simulink subsystem "thermal_basic_peripherals"  (R2023a)
settings: Solver=VariableStepAuto  StartTime=0.0  StopTime=10.0  RelTol=1e-3
values from neighbouring files (symbols this model uses):
  coolant_initial_pressure = 0.111325    [thermal_plant_h2f175_parameters.m]
  coolant_initial_temperature = 293.15    [thermal_plant_h2f175_parameters.m]
  coolant_tube_D = 0.05    [thermal_plant_h2f175_parameters.m]
  tcp_time_constant = 2    [thermal_plant_h2f175_parameters.m]
undefined symbols (not defined in the file or in its folder): air_cp, air_HC_min, air_HC_nom, air_rho, air_vel_nom, radiator_area_air, radiator_area_fins, radiator_area_primary, radiator_n_tubes, radiator_tube_height, radiator_tube_length, radiator_width
libraries: fl_lib x30, nesl_utility x20, SimscapeFluids_lib x5
settings Model: Creator=stefan.notter  LastModifiedBy=stefan.notter

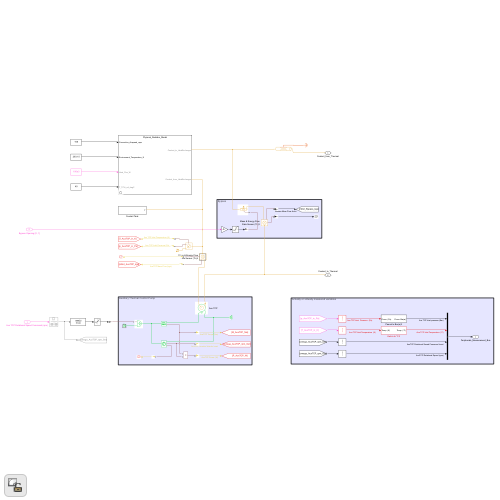
[thumbnail: Simulink's stored preview of the top-level diagram]
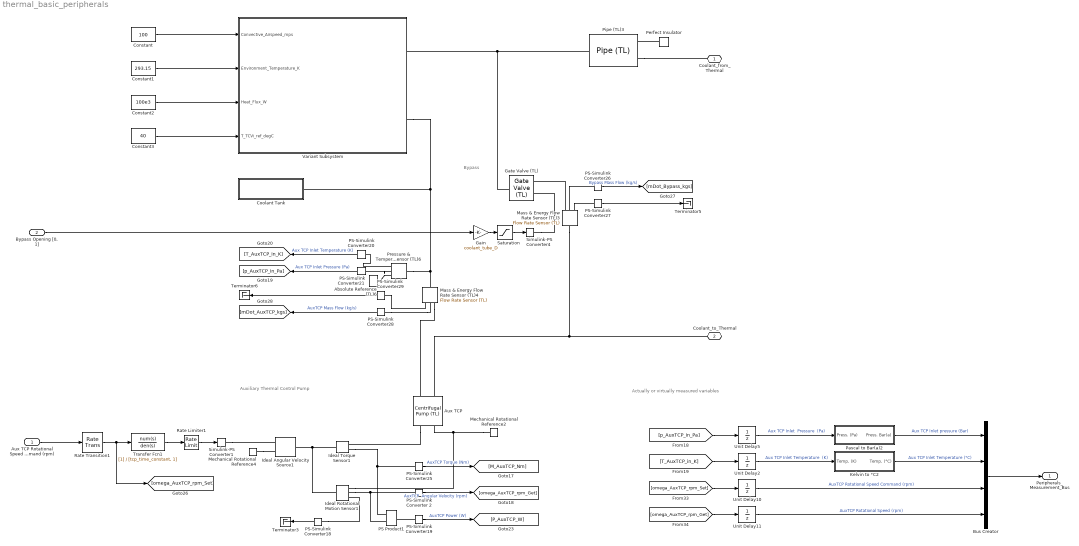
== system thermal_basic_peripherals ==
  note: Auxiliary Thermal Control Pump
  note: Actually or virtually measured variables
  note: Bypass
  Aux TCP Rotational Speed Command (rpm) : Inport
  "Bypass Opening [0, 1]" : Inport  Port=2
  Absolute Reference (TL)6 : fl_lib/Thermal Liquid/Elements/Absolute Reference (TL)
  Aux TCP : SimscapeFluids_lib/Thermal Liquid/Pumps & Motors/Centrifugal Pump (TL)  pump_parameterization=fluids.thermal_liquid.pumps_motors.enum.CentrifugalPumpParameterization.Nominal  capacity_ref_nominal=6000/60 lpm  head_ref_nominal=|  power_ref_nominal=0.3 kW  head_ref_max=|  capacity_ref_max=12000/60 lpm  omega_ref_analytic=3500 rpm  flow_rate_1D_TLU=[1000, 2000, 3000, 4000, 5000, 6000, 7000, 8000, 9000, 1000] lpm  head_1D_TLU=[50, 47.5, 45, 40, 35, 25] m  power_1D_TLU=[.6, .75, .85, .93, .98, .99] kW  omega_ref_1D=3500 rpm  rho_ref_1D=998.21 kg/m^3  omega_threshold_factor=1e-2  flow_rate_2D_TLU=[16.67, 23.33, 30, 40, 53.33, 60] lpm  omega_2D_TLU=[2450, 2800, 3150, 3500] rpm  head_2D_TLU=[25, 32.7, 42.5, 50; 24, 31.7, 41, 49; 22.7, 30.5, 39, 47.5; 20, 28, 36, 45; 15.7, 24, 32, 40; 12.5, 21, 29.5, 37.5] m  power_2D_TLU=[.28, .38, .5, .6; .31, .41, .55, .68; .33, .44, .6, .75; .36, .48, .65, .83; .38, .53, .72, .93; .39, .55, .75, .97] kW  rho_ref_2D=998.21 kg/m^3  diameter_ratio=1  mech_orientation=fluids.thermal_liquid.pumps_motors.enum.CentrifugalPumpMechOrientation.Positive  area=9.6211275016187417927918453612935e-4 m^2
      head_ref_nominal=|
      | 1.2*10^5/(1000*9.81)
      |  m
      head_ref_max=|
      | 1.55*10^5/(1000*9.81)
      |  m
      settings: InternalSimscapePortConfiguration="{\"Bottom\":[],\"Left\":[{\"id\":\"A\",\"label\":\"A\",\"type\":\"foundation.thermal_liquid.thermal_liquid\"},{\"id\":\"B\",\"label\":\"B\",\"type\":\"foundation.thermal_liquid.thermal_liquid\"}],\"Right\":[{\"id\":\"R\",\"label\":\"R\",\"type\":\"foundation.mechanical.rotational.rotational\"},{\"id\":\"C\",\"label\":\"C\",\"type\":\"foundation.mechanical.rotational.rotational\"}],\"Top\":[]}"
  Bus Creator : BusCreator  Inputs=4
  Constant : Constant  Value=100
  Constant1 : Constant  Value=293.15
  Constant2 : Constant  Value=100e3
  Constant3 : Constant  Value=40
  Coolant Tank : Subsystem  Tag=PublishSubsystem  mask(Coolant Tank){A=1, x_init=0.08}
      mask prompts: A "Tank area (m^2)"; x_init "Initial coolant level (m)"
      mask help: This subsystem models an expansion tank for the coolant system.
  Gain : Gain  Gain=coolant_tube_D
  Gate Valve (TL) : SimscapeFluids_lib/Thermal Liquid/Valves & Orifices/Flow Control Valves/Gate Valve (TL)  diam_orifice=coolant_tube_D*0.9 m  S_min=0 m  area_leak=1e-12 m^2  smoothing_factor=0.01  area=pi*coolant_tube_D^2/4 m^2  Cd=0.7  Re_c=12
      settings: InternalSimscapePortConfiguration="{\"Bottom\":[],\"Left\":[{\"id\":\"A\",\"label\":\"A\",\"type\":\"foundation.thermal_liquid.thermal_liquid\"},{\"id\":\"S\",\"label\":\"S\",\"type\":\"input\"}],\"Right\":[{\"id\":\"B\",\"label\":\"B\",\"type\":\"foundation.thermal_liquid.thermal_liquid\"}],\"Top\":[]}"
  Ideal Angular Velocity Source1 : fl_lib/Mechanical/Mechanical Sources/Ideal Angular Velocity Source
  Ideal Rotational Motion Sensor1 : fl_lib/Mechanical/Mechanical Sensors/Ideal Rotational Motion Sensor  reference=foundation.enum.MeasurementReference.difference  acceleration_port=false  velocity_port=true  position_port=true  wrap_angle=false  offset=0 rad
  Ideal Torque Sensor1 : fl_lib/Mechanical/Mechanical Sensors/Ideal Torque Sensor
  Kelvin to °C2 : Subsystem
  Mass & Energy Flow Rate Sensor (TL)3 : fl_lib/Thermal Liquid/Sensors/Flow Rate Sensor (TL)  mass_flow_measure=true  volumetric_flow_measure=false  energy_flow_measure=true
      settings: InternalSimscapePortConfiguration="{\"Bottom\":[{\"id\":\"PHI\",\"label\":\"φ\",\"type\":\"output\"}],\"Left\":[{\"id\":\"A\",\"label\":\"A\",\"type\":\"foundation.thermal_liquid.thermal_liquid\"}],\"Right\":[{\"id\":\"B\",\"label\":\"B\",\"type\":\"foundation.thermal_liquid.thermal_liquid\"},{\"id\":\"M\",\"label\":\"M\",\"type\":\"output\"}],\"Top\":[]}"
  Mass & Energy Flow Rate Sensor (TL)4 : fl_lib/Thermal Liquid/Sensors/Flow Rate Sensor (TL)  mass_flow_measure=true  volumetric_flow_measure=false  energy_flow_measure=true
      settings: InternalSimscapePortConfiguration="{\"Bottom\":[{\"id\":\"PHI\",\"label\":\"φ\",\"type\":\"output\"}],\"Left\":[{\"id\":\"A\",\"label\":\"A\",\"type\":\"foundation.thermal_liquid.thermal_liquid\"}],\"Right\":[{\"id\":\"B\",\"label\":\"B\",\"type\":\"foundation.thermal_liquid.thermal_liquid\"},{\"id\":\"M\",\"label\":\"M\",\"type\":\"output\"}],\"Top\":[]}"
  Mechanical Rotational Reference2 : fl_lib/Mechanical/Rotational Elements/Mechanical Rotational Reference
  Mechanical Rotational Reference4 : fl_lib/Mechanical/Rotational Elements/Mechanical Rotational Reference
  PS Product1 : fl_lib/Physical Signals/Functions/PS Product
  PS-Simulink Converter 2 : nesl_utility/PS-Simulink Converter  PhysicalDomain=network_engine_domain  SubClassName=ps_output  LeftPortType=input  RightPortType=output  PseudoPeriodic=off  Frequencies=[]  VectorFormat=1-D array  Unit=rpm  AffineConversion=off
  PS-Simulink Converter{18,20..21,26..29} (7 alike) : nesl_utility/PS-Simulink Converter  PhysicalDomain=network_engine_domain  SubClassName=ps_output  LeftPortType=input  RightPortType=output  PseudoPeriodic=off  Frequencies=[]  VectorFormat=inherit  Unit=inherit  AffineConversion=off
  PS-Simulink Converter19 : nesl_utility/PS-Simulink Converter  PhysicalDomain=network_engine_domain  SubClassName=ps_output  LeftPortType=input  RightPortType=output  PseudoPeriodic=off  Frequencies=[]  VectorFormat=inherit  Unit=W  AffineConversion=off
  PS-Simulink Converter25 : nesl_utility/PS-Simulink Converter  PhysicalDomain=network_engine_domain  SubClassName=ps_output  LeftPortType=input  RightPortType=output  PseudoPeriodic=off  Frequencies=[]  VectorFormat=inherit  Unit=N*m  AffineConversion=off
  Pascal to Bar(a)2 : Subsystem
  Perfect Insulator : fl_lib/Thermal/Thermal Elements/Perfect Insulator  T_specify=off  T_priority=None  T=293.15 K  T_nominal_specify=off  T_nominal_unit=K  T_nominal_value=1
  Pipe (TL)3 : fl_lib/Thermal Liquid/Elements/Pipe (TL)  length=1 m  area=pi*coolant_tube_D^2/4 m^2  Dh=pi*coolant_tube_D*0.9 m  length_add=1 m  roughness=15e-6 m  Re_lam=2000  Re_tur=4000  shape_factor=64  Nu_lam=3.66  dynamic_compressibility=simscape.enum.onoff.on  inertia=simscape.enum.onoff.off  p0=coolant_initial_pressure MPa  T0=coolant_initial_temperature K  mdot0=0 kg/s
  Pressure & Temperature Sensor (TL)6 : fl_lib/Thermal Liquid/Sensors/Pressure & Temperature Sensor (TL)  reference=foundation.enum.MeasurementReference.difference  pressure=true  pressure_spec=foundation.enum.PressureMeasementSpec.Absolute  temperature=true
      settings: InternalSimscapePortConfiguration="{\"Bottom\":[{\"id\":\"T\",\"label\":\"T\",\"type\":\"output\"}],\"Left\":[{\"id\":\"A\",\"label\":\"A\",\"type\":\"foundation.thermal_liquid.thermal_liquid\"}],\"Right\":[{\"id\":\"B\",\"label\":\"B\",\"type\":\"foundation.thermal_liquid.thermal_liquid\"},{\"id\":\"P\",\"label\":\"P\",\"type\":\"output\"}],\"Top\":[]}"
  Rate Limiter1 : RateLimiter  RisingSlewLimit=1000  FallingSlewLimit=-1000  SampleTimeMode=inherited
  Rate Transition1 : RateTransition
  Saturation : Saturate  UpperLimit=coolant_tube_D  LowerLimit=0
  Simulink-PS Converter1 : nesl_utility/Simulink-PS Converter  PhysicalDomain=network_engine_domain  SubClassName=ps_input  LeftPortType=input  RightPortType=output  PseudoPeriodic=off  Frequencies=[]  NoiseDistribution=none  NoiseParameters=[]  Unit=rpm  AffineConversion=off  FilteringAndDerivatives=provide  SimscapeFilterOrder=1  InputFilterTimeConstant=0.001  UdotUserProvided=0
  Simulink-PS Converter4 : nesl_utility/Simulink-PS Converter  PhysicalDomain=network_engine_domain  SubClassName=ps_input  LeftPortType=input  RightPortType=output  PseudoPeriodic=off  Frequencies=[]  NoiseDistribution=none  NoiseParameters=[]  Unit=1  AffineConversion=off  FilteringAndDerivatives=provide  SimscapeFilterOrder=1  InputFilterTimeConstant=0.001  UdotUserProvided=0
  Terminator3 : Terminator
  Terminator5 : Terminator
  Terminator6 : Terminator
  Transfer Fcn1 : TransferFcn  Denominator=[tcp_time_constant, 1]  ContinuousStateAttributes='tcv_opening'
  Unit Delay10 : UnitDelay  SampleTime=-1  HasFrameUpgradeWarning=on
  Unit Delay11 : UnitDelay  SampleTime=-1  HasFrameUpgradeWarning=on
  Unit Delay2 : UnitDelay  InitialCondition=coolant_initial_temperature  SampleTime=-1  HasFrameUpgradeWarning=on
  Unit Delay5 : UnitDelay  InitialCondition=coolant_initial_pressure  SampleTime=-1  HasFrameUpgradeWarning=on
  Variant Subsystem : Subsystem  Variant=on
  Coolant_from_Thermal : PMIOPort  Side=Left
  Coolant_to_Thermal : PMIOPort  Port=2  Side=Left
  Peripherals_Measurement_Bus : Outport
  wires:
  Aux TCP Rotational Speed Command (rpm)/1 -> Rate Transition1/1
  PS-Simulink Converter29/1 -> Terminator6/1
  PS-Simulink Converter20/1 -> [T_AuxTCP_in_K]  "Aux TCP Inlet Temperature (K)"
  PS-Simulink Converter21/1 -> [p_AuxTCP_in_Pa]  "Aux TCP Inlet Pressure (Pa)"
  PS-Simulink Converter19/1 -> [P_AuxTCP_W]  "AuxTCP Power (W)"
  Rate Transition1/1 -> Transfer Fcn1/1, [omega_AuxTCP_rpm_Set]
  PS-Simulink Converter 2/1 -> [omega_AuxTCP_rpm_Get]  "AuxTCP  Angular Velocity (rpm)"
  PS-Simulink Converter25/1 -> [M_AuxTCP_Nm]  "AuxTCP Torque (Nm)"
  PS-Simulink Converter18/1 -> Terminator3/1
  Rate Limiter1/1 -> Simulink-PS Converter1/1
  Transfer Fcn1/1 -> Rate Limiter1/1
  PS-Simulink Converter28/1 -> [mDot_AuxTCP_kgs]  "AuxTCP Mass Flow (kg/s)"
  Pascal to Bar(a)2/1(Press. Bar(a)) -> Bus Creator/1  "Aux TCP Inlet pressure (Bar)"
  Unit Delay10/1 -> Bus Creator/3  "AuxTCP Rotational Speed Command (rpm)"
  Kelvin to °C2/1(Temp. (°C)) -> Bus Creator/2  "Aux TCP Inlet Temperature (°C)"
  [omega_AuxTCP_rpm_Get] -> Unit Delay11/1
  Unit Delay2/1 -> Kelvin to °C2/1(Temp. (K))  "Aux TCP Inlet Temperature  (K)"
  Unit Delay5/1 -> Pascal to Bar(a)2/1(Press. (Pa))  "Aux TCP Inlet  Pressure  (Pa)"
  Unit Delay11/1 -> Bus Creator/4  "AuxTCP Rotational Speed (rpm)"
  [p_AuxTCP_in_Pa] -> Unit Delay5/1
  [T_AuxTCP_in_K] -> Unit Delay2/1
  [omega_AuxTCP_rpm_Set] -> Unit Delay10/1
  Bus Creator/1 -> Peripherals_Measurement_Bus/1
  Constant/1 -> Variant Subsystem/1(Convective_Airspeed_mps)
  Constant1/1 -> Variant Subsystem/2(Environment_Temperature_K)
  Constant2/1 -> Variant Subsystem/3(Heat_Flux_W)
  Constant3/1 -> Variant Subsystem/4(T_TCVi_ref_degC)
  PS-Simulink Converter26/1 -> [mDot_Bypass_kgs]  "Bypass Mass Flow (kg/s)"
  PS-Simulink Converter27/1 -> Terminator5/1
  Gain/1 -> Saturation/1
  "Bypass Opening [0, 1]"/1 -> Gain/1
  Saturation/1 -> Simulink-PS Converter4/1
  connections:
  Mechanical Rotational Reference2/LConn1 -- Aux TCP/RConn2 -- Ideal Rotational Motion Sensor1/RConn1
  Variant Subsystem/RConn2 -- Coolant Tank/RConn1 -- Mass & Energy Flow Rate Sensor (TL)4/LConn1 -- Pressure & Temperature Sensor (TL)6/LConn1
  Ideal Angular Velocity Source1/LConn1 -- Ideal Rotational Motion Sensor1/LConn1 -- Ideal Torque Sensor1/LConn1
  Ideal Rotational Motion Sensor1/RConn2 -- PS Product1/LConn2 -- PS-Simulink Converter 2/LConn1
  Ideal Torque Sensor1/RConn2 -- PS-Simulink Converter25/LConn1 -- PS Product1/LConn1
  Aux TCP/LConn2 -- Coolant_to_Thermal/RConn1 -- Mass & Energy Flow Rate Sensor (TL)3/LConn1
  Gate Valve (TL)/RConn1 -- Variant Subsystem/RConn1 -- Pipe (TL)3/RConn1
  Simulink-PS Converter1/RConn1 -- Ideal Angular Velocity Source1/RConn1
  PS-Simulink Converter28/LConn1 -- Mass & Energy Flow Rate Sensor (TL)4/RConn2
  Pressure & Temperature Sensor (TL)6/RConn1 -- Absolute Reference (TL)6/LConn1
  Pressure & Temperature Sensor (TL)6/RConn2 -- PS-Simulink Converter21/LConn1
  Aux TCP/RConn1 -- Ideal Torque Sensor1/RConn1
  Mechanical Rotational Reference4/LConn1 -- Ideal Angular Velocity Source1/RConn2
  PS-Simulink Converter18/LConn1 -- Ideal Rotational Motion Sensor1/RConn3
  PS-Simulink Converter19/LConn1 -- PS Product1/RConn1
  Mass & Energy Flow Rate Sensor (TL)4/RConn1 -- Aux TCP/LConn1
  Pressure & Temperature Sensor (TL)6/RConn3 -- PS-Simulink Converter20/LConn1
  PS-Simulink Converter29/LConn1 -- Mass & Energy Flow Rate Sensor (TL)4/RConn3
  Mass & Energy Flow Rate Sensor (TL)3/RConn1 -- Gate Valve (TL)/LConn1
  PS-Simulink Converter26/LConn1 -- Mass & Energy Flow Rate Sensor (TL)3/RConn2
  Simulink-PS Converter4/RConn1 -- Gate Valve (TL)/LConn2
  PS-Simulink Converter27/LConn1 -- Mass & Energy Flow Rate Sensor (TL)3/RConn3
  Pipe (TL)3/LConn1 -- Coolant_from_Thermal/RConn1
  Perfect Insulator/LConn1 -- Pipe (TL)3/LConn2

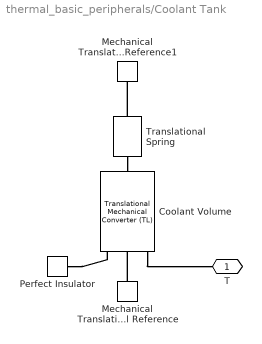
== system thermal_basic_peripherals/Coolant Tank ==
  Coolant Volume : fl_lib/Thermal Liquid/Elements/Translational Mechanical Converter (TL)  mech_orientation=foundation.enum.MechOrientationTranslational.Positive  displacement_spec=foundation.enum.DisplacementSpec.Calculate  x0=x_init m  interface_area=A m^2  dead_volume=A * 0.001 m^3  environment_spec=foundation.enum.pressure_spec.specified  environment_pressure=coolant_initial_pressure MPa  dynamic_compressibility=simscape.enum.onoff.off  p0=env_p MPa  T0=coolant_initial_temperature K
      settings: InternalSimscapePortConfiguration="{\"Bottom\":[],\"Left\":[{\"id\":\"A\",\"label\":\"A\",\"type\":\"foundation.thermal_liquid.thermal_liquid\"},{\"id\":\"C\",\"label\":\"C\",\"type\":\"foundation.mechanical.translational.translational\"},{\"id\":\"H\",\"label\":\"H\",\"type\":\"foundation.thermal.thermal\"}],\"Right\":[{\"id\":\"R\",\"label\":\"R\",\"type\":\"foundation.mechanical.translational.translational\"}],\"Top\":[]}"
  Mechanical Translational Reference : fl_lib/Mechanical/Translational Elements/Mechanical Translational Reference
  Mechanical Translational Reference1 : fl_lib/Mechanical/Translational Elements/Mechanical Translational Reference
  Perfect Insulator : fl_lib/Thermal/Thermal Elements/Perfect Insulator  T_specify=off  T_priority=None  T=0 K  T_nominal_specify=off  T_nominal_unit=K  T_nominal_value=1
  Translational Spring : fl_lib/Mechanical/Translational Elements/Translational Spring  spr_rate=1e6 N/m  v_specify=off  v_priority=None  v=0 m/s  v_nominal_specify=off  v_nominal_unit=m/s  v_nominal_value=1  f_specify=off  f_priority=None  f=0 N  f_nominal_specify=off  f_nominal_unit=N  f_nominal_value=1  x_specify=off  x_priority=High  x=x_init m  x_nominal_specify=on  x_nominal_unit=m  x_nominal_value=x_init
  T : PMIOPort  Side=Right
  connections:
  Translational Spring/LConn1 -- Mechanical Translational Reference1/LConn1
  Translational Spring/RConn1 -- Coolant Volume/RConn1
  Perfect Insulator/LConn1 -- Coolant Volume/LConn3
  Mechanical Translational Reference/LConn1 -- Coolant Volume/LConn2
  Coolant Volume/LConn1 -- T/RConn1

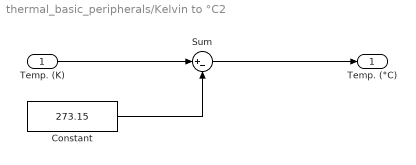
== system thermal_basic_peripherals/Kelvin to °C2 ==
  Temp. (K) : Inport
  Constant : Constant  Value=273.15
  Sum : Sum  Inputs=|+-
  Temp. (°C) : Outport
  wires:
  Temp. (K)/1 -> Sum/1
  Sum/1 -> Temp. (°C)/1
  Constant/1 -> Sum/2

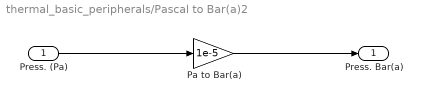
== system thermal_basic_peripherals/Pascal to Bar(a)2 ==
  Press. (Pa) : Inport
  Pa to Bar(a) : Gain  Gain=1e-5
  Press. Bar(a) : Outport
  wires:
  Press. (Pa)/1 -> Pa to Bar(a)/1
  Pa to Bar(a)/1 -> Press. Bar(a)/1

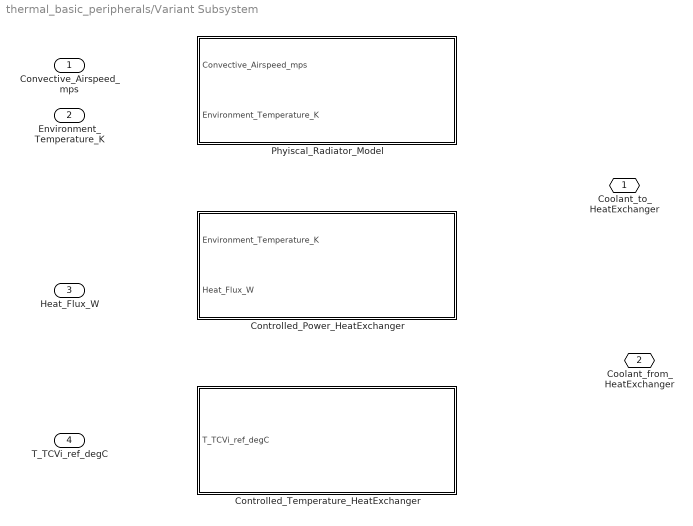
== system thermal_basic_peripherals/Variant Subsystem ==
  Convective_Airspeed_mps : Inport
  Environment_Temperature_K : Inport  Port=2
  Heat_Flux_W : Inport  Port=3
  T_TCVi_ref_degC : Inport  Port=4
  Controlled_Power_HeatExchanger : Subsystem  VariantControl=HEATEXCHANGER_VARIANT_POWER_CONTROLLED
  Controlled_Temperature_HeatExchanger : Subsystem  VariantControl=HEATEXCHANGER_VARIANT_TEMP_CONTROLLED
  Phyiscal_Radiator_Model : Subsystem  VariantControl=HEATEXCHANGER_VARIANT_PHYSICAL
  Coolant_to_HeatExchanger : PMIOPort  Side=Right
  Coolant_from_HeatExchanger : PMIOPort  Port=2  Side=Right

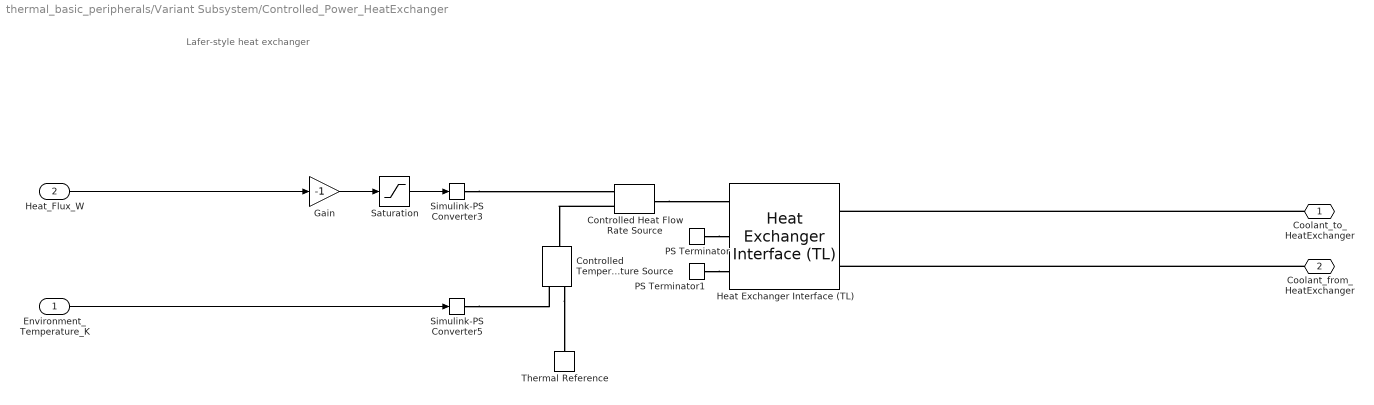
== system thermal_basic_peripherals/Variant Subsystem/Controlled_Power_HeatExchanger ==
  note: Lafer-style heat exchanger
  Environment_Temperature_K : Inport
  Heat_Flux_W : Inport  Port=2
  Controlled Temperature Source : fl_lib/Thermal/Thermal Sources/Controlled Temperature Source
  Controlled Heat Flow Rate Source : fl_lib/Thermal/Thermal Sources/Controlled Heat Flow Rate Source
  Gain : Gain  Gain=-1
  Heat Exchanger Interface (TL) : SimscapeFluids_lib/Fluid Network Interfaces/Heat Exchangers/Fundamental Components/Heat Exchanger Interface (TL)  min_flow_area=radiator_n_tubes*(radiator_width*radiator_tube_height) m^2  Dh_press=4*(radiator_width*radiator_tube_height)/(2 * (radiator_width+radiator_tube_height)) m  liquid_volume=radiator_n_tubes*(radiator_width*radiator_tube_height)*radiator_tube_length m^3  Re_lam=2000  Re_tur=4000.  pressure_loss_spec=fluids.interfaces.enum.pressure_loss_spec.tube_correlation  pressure_loss_coeff=0.1  length_press=radiator_tube_length m  length_add=0.1 m  roughness=15e-6 m  Re_friction_TLU=[400, 1000, 1500, 3000, 4000, 6000, 10000, 20000, 40000, 60000, 100000, 100000000]  friction_factor_TLU=[.264, .112, .071, .0417, .0387, .0268, .025, .0232, .0226, .022, .0214, .0214]  shape_factor=64  Re_Euler_TLU=[50, 500, 1000, 2000]  Euler_TLU=[4.4505, .6864, .4791, .3755]  heat_transfer_spec=fluids.interfaces.enum.heat_transfer_spec.tube_correlation  heat_coeff=100 W/(K*m^2)  heat_transfer_area=radiator_n_tubes*2*(radiator_tube_length*radiator_width+radiator_tube_length*radiator_tube_height) m^2  Nu_lam=3.66  Re_Colburn_TLU=[100, 150, 1000]  Colburn_factor_TLU=[.019, .013, .002]  Re_Nu_TLU=[100, 150, 1000]  Pr_Nu_TLU=[1, 10]  Nu_TLU=[3.72, 4.21; 3.75, 4.44; 4.21, 7.15]  length_heat=radiator_tube_length m  dynamic_compressibility=simscape.enum.onoff.on  T0=coolant_initial_temperature K  p0=coolant_initial_pressure MPa
      settings: InternalSimscapePortConfiguration="{\"Bottom\":[],\"Left\":[{\"id\":\"A\",\"label\":\"A\",\"type\":\"foundation.thermal_liquid.thermal_liquid\"},{\"id\":\"B\",\"label\":\"B\",\"type\":\"foundation.thermal_liquid.thermal_liquid\"}],\"Right\":[{\"id\":\"H\",\"label\":\"H\",\"type\":\"foundation.thermal.thermal\"},{\"id\":\"C\",\"label\":\"C\",\"type\":\"output\"},{\"id\":\"HC\",\"label\":\"HC\",\"type\":\"output\"}],\"Top\":[]}"
  PS Terminator : fl_lib/Physical Signals/Sinks/PS Terminator
  PS Terminator1 : fl_lib/Physical Signals/Sinks/PS Terminator
  Saturation : Saturate  UpperLimit=0  LowerLimit=-200e3
  Simulink-PS Converter3 : nesl_utility/Simulink-PS Converter  PhysicalDomain=network_engine_domain  SubClassName=ps_input  LeftPortType=input  RightPortType=output  PseudoPeriodic=off  Frequencies=[]  NoiseDistribution=none  NoiseParameters=[]  Unit=1  AffineConversion=off  FilteringAndDerivatives=provide  SimscapeFilterOrder=1  InputFilterTimeConstant=0.001  UdotUserProvided=0
  Simulink-PS Converter5 : nesl_utility/Simulink-PS Converter  PhysicalDomain=network_engine_domain  SubClassName=ps_input  LeftPortType=input  RightPortType=output  PseudoPeriodic=off  Frequencies=[]  NoiseDistribution=none  NoiseParameters=[]  Unit=1  AffineConversion=off  FilteringAndDerivatives=provide  SimscapeFilterOrder=1  InputFilterTimeConstant=0.001  UdotUserProvided=0
  Thermal Reference : fl_lib/Thermal/Thermal Elements/Thermal Reference
  Coolant_to_HeatExchanger : PMIOPort  Side=Right
  Coolant_from_HeatExchanger : PMIOPort  Port=2  Side=Right
  wires:
  Saturation/1 -> Simulink-PS Converter3/1
  Gain/1 -> Saturation/1
  Heat_Flux_W/1 -> Gain/1
  Environment_Temperature_K/1 -> Simulink-PS Converter5/1
  connections:
  Coolant_from_HeatExchanger/RConn1 -- Heat Exchanger Interface (TL)/LConn2
  Simulink-PS Converter5/RConn1 -- Controlled Temperature Source/RConn1
  PS Terminator1/LConn1 -- Heat Exchanger Interface (TL)/RConn3
  Simulink-PS Converter3/RConn1 -- Controlled Heat Flow Rate Source/RConn1
  Controlled Heat Flow Rate Source/LConn1 -- Heat Exchanger Interface (TL)/RConn1
  Controlled Temperature Source/RConn2 -- Thermal Reference/LConn1
  Controlled Heat Flow Rate Source/RConn2 -- Controlled Temperature Source/LConn1
  PS Terminator/LConn1 -- Heat Exchanger Interface (TL)/RConn2
  Coolant_to_HeatExchanger/RConn1 -- Heat Exchanger Interface (TL)/LConn1

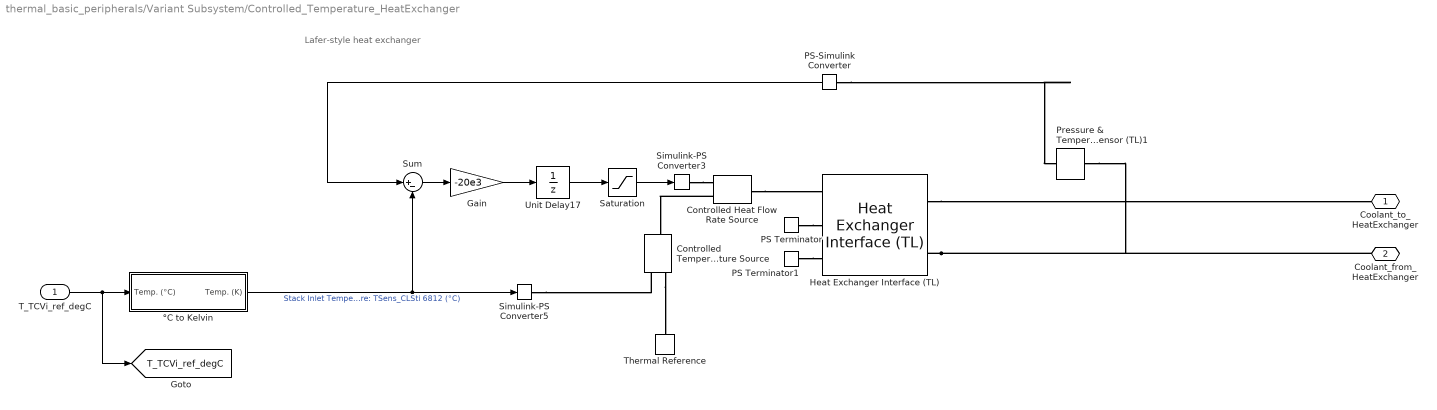
== system thermal_basic_peripherals/Variant Subsystem/Controlled_Temperature_HeatExchanger ==
  note: Lafer-style heat exchanger
  T_TCVi_ref_degC : Inport
  Controlled Temperature Source : fl_lib/Thermal/Thermal Sources/Controlled Temperature Source
  Controlled Heat Flow Rate Source : fl_lib/Thermal/Thermal Sources/Controlled Heat Flow Rate Source
  Gain : Gain  Gain=-20e3
  Heat Exchanger Interface (TL) : SimscapeFluids_lib/Fluid Network Interfaces/Heat Exchangers/Fundamental Components/Heat Exchanger Interface (TL)  min_flow_area=radiator_n_tubes*(radiator_width*radiator_tube_height) m^2  Dh_press=4*(radiator_width*radiator_tube_height)/(2 * (radiator_width+radiator_tube_height)) m  liquid_volume=radiator_n_tubes*(radiator_width*radiator_tube_height)*radiator_tube_length m^3  Re_lam=2000  Re_tur=4000.  pressure_loss_spec=fluids.interfaces.enum.pressure_loss_spec.tube_correlation  pressure_loss_coeff=0.1  length_press=radiator_tube_length m  length_add=0.1 m  roughness=15e-6 m  Re_friction_TLU=[400, 1000, 1500, 3000, 4000, 6000, 10000, 20000, 40000, 60000, 100000, 100000000]  friction_factor_TLU=[.264, .112, .071, .0417, .0387, .0268, .025, .0232, .0226, .022, .0214, .0214]  shape_factor=64  Re_Euler_TLU=[50, 500, 1000, 2000]  Euler_TLU=[4.4505, .6864, .4791, .3755]  heat_transfer_spec=fluids.interfaces.enum.heat_transfer_spec.tube_correlation  heat_coeff=100 W/(K*m^2)  heat_transfer_area=radiator_n_tubes*2*(radiator_tube_length*radiator_width+radiator_tube_length*radiator_tube_height) m^2  Nu_lam=3.66  Re_Colburn_TLU=[100, 150, 1000]  Colburn_factor_TLU=[.019, .013, .002]  Re_Nu_TLU=[100, 150, 1000]  Pr_Nu_TLU=[1, 10]  Nu_TLU=[3.72, 4.21; 3.75, 4.44; 4.21, 7.15]  length_heat=radiator_tube_length m  dynamic_compressibility=simscape.enum.onoff.on  T0=coolant_initial_temperature K  p0=coolant_initial_pressure MPa
      settings: InternalSimscapePortConfiguration="{\"Bottom\":[],\"Left\":[{\"id\":\"A\",\"label\":\"A\",\"type\":\"foundation.thermal_liquid.thermal_liquid\"},{\"id\":\"B\",\"label\":\"B\",\"type\":\"foundation.thermal_liquid.thermal_liquid\"}],\"Right\":[{\"id\":\"H\",\"label\":\"H\",\"type\":\"foundation.thermal.thermal\"},{\"id\":\"C\",\"label\":\"C\",\"type\":\"output\"},{\"id\":\"HC\",\"label\":\"HC\",\"type\":\"output\"}],\"Top\":[]}"
  PS Terminator : fl_lib/Physical Signals/Sinks/PS Terminator
  PS Terminator1 : fl_lib/Physical Signals/Sinks/PS Terminator
  PS-Simulink Converter : nesl_utility/PS-Simulink Converter  PhysicalDomain=network_engine_domain  SubClassName=ps_output  LeftPortType=input  RightPortType=output  PseudoPeriodic=off  Frequencies=[]  VectorFormat=inherit  Unit=inherit  AffineConversion=off
  Pressure & Temperature Sensor (TL)1 : fl_lib/Thermal Liquid/Sensors/Pressure & Temperature Sensor (TL)  reference=foundation.enum.MeasurementReference.absolute  pressure=false  pressure_spec=foundation.enum.PressureMeasementSpec.Absolute  temperature=true
      settings: InternalSimscapePortConfiguration="{\"Bottom\":[{\"id\":\"T\",\"label\":\"T\",\"type\":\"output\"}],\"Left\":[{\"id\":\"A\",\"label\":\"A\",\"type\":\"foundation.thermal_liquid.thermal_liquid\"}],\"Right\":[],\"Top\":[]}"
  Saturation : Saturate  UpperLimit=0  LowerLimit=-200e3
  Simulink-PS Converter3 : nesl_utility/Simulink-PS Converter  PhysicalDomain=network_engine_domain  SubClassName=ps_input  LeftPortType=input  RightPortType=output  PseudoPeriodic=off  Frequencies=[]  NoiseDistribution=none  NoiseParameters=[]  Unit=1  AffineConversion=off  FilteringAndDerivatives=provide  SimscapeFilterOrder=1  InputFilterTimeConstant=0.001  UdotUserProvided=0
  Simulink-PS Converter5 : nesl_utility/Simulink-PS Converter  PhysicalDomain=network_engine_domain  SubClassName=ps_input  LeftPortType=input  RightPortType=output  PseudoPeriodic=off  Frequencies=[]  NoiseDistribution=none  NoiseParameters=[]  Unit=1  AffineConversion=off  FilteringAndDerivatives=provide  SimscapeFilterOrder=1  InputFilterTimeConstant=0.001  UdotUserProvided=0
  Sum : Sum  Inputs=|+-
  Thermal Reference : fl_lib/Thermal/Thermal Elements/Thermal Reference
  Unit Delay17 : UnitDelay  SampleTime=-1  HasFrameUpgradeWarning=on
  °C to Kelvin : Subsystem
  Coolant_to_HeatExchanger : PMIOPort  Side=Right
  Coolant_from_HeatExchanger : PMIOPort  Port=2  Side=Right
  tag scope: T_TCVi_ref_degC=global
  wires:
  °C to Kelvin/1(Temp. (K)) -> Sum/2, Simulink-PS Converter5/1  "Stack Inlet Temperature: TSens_CLSti 6812 (°C)"
  Saturation/1 -> Simulink-PS Converter3/1
  Sum/1 -> Gain/1
  T_TCVi_ref_degC/1 -> °C to Kelvin/1(Temp. (°C)), [T_TCVi_ref_degC]
  Unit Delay17/1 -> Saturation/1
  Gain/1 -> Unit Delay17/1
  PS-Simulink Converter/1 -> Sum/1
  connections:
  Heat Exchanger Interface (TL)/LConn1 -- Coolant_to_HeatExchanger/RConn1
  PS Terminator/LConn1 -- Heat Exchanger Interface (TL)/RConn2
  Controlled Heat Flow Rate Source/RConn2 -- Controlled Temperature Source/LConn1
  PS-Simulink Converter/LConn1 -- Pressure & Temperature Sensor (TL)1/RConn1
  Controlled Temperature Source/RConn2 -- Thermal Reference/LConn1
  Controlled Heat Flow Rate Source/LConn1 -- Heat Exchanger Interface (TL)/RConn1
  Simulink-PS Converter3/RConn1 -- Controlled Heat Flow Rate Source/RConn1
  PS Terminator1/LConn1 -- Heat Exchanger Interface (TL)/RConn3
  Simulink-PS Converter5/RConn1 -- Controlled Temperature Source/RConn1
  Heat Exchanger Interface (TL)/LConn2 -- Pressure & Temperature Sensor (TL)1/LConn1 -- Coolant_from_HeatExchanger/RConn1

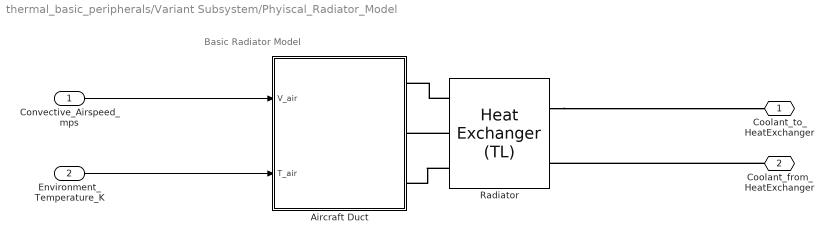
== system thermal_basic_peripherals/Variant Subsystem/Phyiscal_Radiator_Model ==
  note: Basic Radiator Model
  Convective_Airspeed_mps : Inport
  Environment_Temperature_K : Inport  Port=2
  Aircraft Duct : Subsystem
  Radiator : SimscapeFluids_lib/Fluid Network Interfaces/Heat Exchangers/Heat Exchanger (TL)  hex_type=3  shell_num=1  cross_type=4  NTU_TLU=[0.5, 1.0, 2.0, 3.0, 4.0, 5.0]  CR_TLU=[0.0, 0.25, 0.5, 0.75, 1.0]  eff_TLU=[0.3, 0.3, 0.3, 0.3, 0.3; 0.6, 0.55, 0.5, 0.47, 0.43; 0.85, 0.76, 0.68, 0.61, 0.55; 0.94, 0.83, 0.72, 0.65, 0.58; 0.98, 0.86, 0.75, 0.66, 0.58; 0.99, 0.86, 0.75, 0.66, 0.58]  R_wall=0.014/(381*radiator_n_tubes*radiator_width*radiator_tube_length) K/W  min_flow_area_1=radiator_n_tubes*(radiator_width*radiator_tube_height) m^2  Dh_press_1=4*(radiator_width*radiator_tube_height)/(2 * (radiator_width+radiator_tube_height)) m  liquid_volume_1=radiator_n_tubes*(radiator_width*radiator_tube_height)*radiator_tube_length m^3  Re_lam_1=2000  Re_tur_1=4000  pressure_loss_spec_1=fluids.interfaces.enum.pressure_loss_spec.tube_correlation  pressure_loss_coeff_1=15  length_press_1=radiator_tube_length m  length_add_1=0.1 m  roughness_1=15e-6 m  Re_friction_TLU_1=[400.0, 1000.0, 1500.0, 3000.0, 4000.0, 6000.0, 10000.0, 20000.0, 40000.0, 60000.0, 100000.0, 100000000.0]  friction_factor_TLU_1=[0.264, 0.112, 0.071, 0.0417, 0.0387, 0.0268, 0.025, 0.0232, 0.0226, 0.022, 0.0214, 0.0214]  shape_factor_1=64  Re_Euler_TLU_1=[50.0, 500.0, 1000.0, 2000.0]  Euler_TLU_1=[4.4505, 0.6864, 0.4791, 0.3755]  heat_transfer_spec_1=2  heat_transfer_area_1=radiator_n_tubes*2*(radiator_tube_length*radiator_width+radiator_tube_length*radiator_tube_height) m^2  heat_coeff_1=2000 W/(m^2 * K)  length_heat_1=radiator_tube_length cm  Nu_lam_1=3.66  Re_Colburn_TLU_1=[100.0, 150.0, 1000.0]  Colburn_factor_TLU_1=[0.019, 0.013, 0.002]  Re_Nu_TLU_1=[100.0, 150.0, 1000.0]  Pr_Nu_TLU_1=[1.0, 10.0]  Nu_TLU_1=[3.72, 4.21; 3.75, 4.44; 4.21, 7.15]  fouling_factor_1=0 m^2*K/W  min_heat_coeff_1=5 W/(m^2 * K)  heat_transfer_area_2=radiator_area_primary+radiator_area_fins m^2  fouling_factor_2=0 m^2*K/W  min_heat_coeff_2=0.01 W/(m^2 * K)  dynamic_compressibility_1=1  T0_1=coolant_initial_temperature K  p0_1=coolant_initial_pressure MPa  mdot1_TLU=[.1, .2] kg/s  mdot2_TLU=[.2, .3] kg/s  SD_TLU=[35, 35; 50, 50] kW/K  Q_check=1  mdot_dp_TLU_1=[.1, .2] kg/s  p_diff_TLU_1=[.003, .005] MPa  T_ref_in_1=293.15 K  p_ref_in_1=0.101325 MPa  mdot_threshold_1=1e-3 kg/s  area_1=0.01 m^2
      settings: InternalSimscapePortConfiguration="{\"Bottom\":[],\"Left\":[{\"id\":\"A1\",\"label\":\"A1\",\"type\":\"foundation.thermal_liquid.thermal_liquid\"},{\"id\":\"B1\",\"label\":\"B1\",\"type\":\"foundation.thermal_liquid.thermal_liquid\"}],\"Right\":[{\"id\":\"H2\",\"label\":\"H2\",\"type\":\"foundation.thermal.thermal\"},{\"id\":\"C2\",\"label\":\"C2\",\"type\":\"input\"},{\"id\":\"HC2\",\"label\":\"HC2\",\"type\":\"input\"}],\"Top\":[]}"
  Coolant_to_HeatExchanger : PMIOPort  Side=Right
  Coolant_from_HeatExchanger : PMIOPort  Port=2  Side=Right
  wires:
  Convective_Airspeed_mps/1 -> Aircraft Duct/1(V_air)
  Environment_Temperature_K/1 -> Aircraft Duct/2(T_air)
  connections:
  Coolant_from_HeatExchanger/RConn1 -- Radiator/LConn2
  Radiator/RConn3 -- Aircraft Duct/RConn3
  Radiator/LConn1 -- Coolant_to_HeatExchanger/RConn1
  Radiator/RConn2 -- Aircraft Duct/RConn2
  Radiator/RConn1 -- Aircraft Duct/RConn1

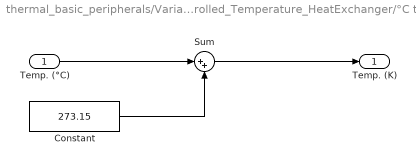
== system thermal_basic_peripherals/Variant Subsystem/Controlled_Temperature_HeatExchanger/°C to Kelvin ==
  Temp. (°C) : Inport
  Constant : Constant  Value=273.15
  Sum : Sum  Inputs=|++
  Temp. (K) : Outport
  wires:
  Temp. (°C)/1 -> Sum/1
  Sum/1 -> Temp. (K)/1
  Constant/1 -> Sum/2

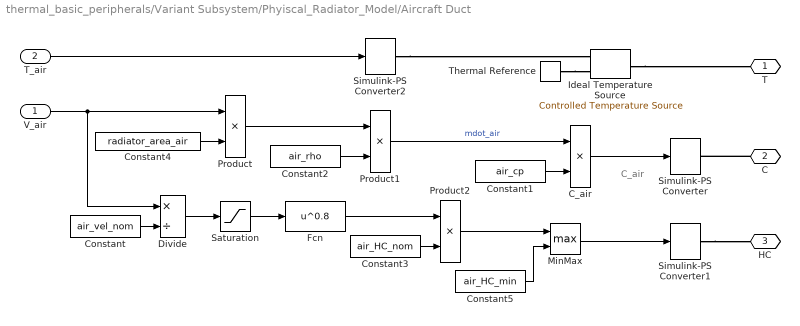
== system thermal_basic_peripherals/Variant Subsystem/Phyiscal_Radiator_Model/Aircraft Duct ==
  note: C_air
  V_air : Inport
  T_air : Inport  Port=2
  C_air : Product
  Constant : Constant  Value=air_vel_nom
  Constant1 : Constant  Value=air_cp
  Constant2 : Constant  Value=air_rho
  Constant3 : Constant  Value=air_HC_nom
  Constant4 : Constant  Value=radiator_area_air
  Constant5 : Constant  Value=air_HC_min
  Divide : Product  Inputs=*/
  Fcn : Fcn  Expr=u^0.8
  Ideal Temperature Source : fl_lib/Thermal/Thermal Sources/Controlled Temperature Source
  MinMax : MinMax  Function=max  Inputs=2
  Product : Product
  Product1 : Product
  Product2 : Product
  Saturation : Saturate  UpperLimit=inf  LowerLimit=0
  Simulink-PS Converter : nesl_utility/Simulink-PS Converter  PhysicalDomain=network_engine_domain  SubClassName=ps_input  LeftPortType=input  RightPortType=output  PseudoPeriodic=off  Frequencies=[]  NoiseDistribution=none  NoiseParameters=[]  Unit=W/K  AffineConversion=off  FilteringAndDerivatives=zero  SimscapeFilterOrder=1  InputFilterTimeConstant=1  UdotUserProvided=1
  Simulink-PS Converter1 : nesl_utility/Simulink-PS Converter  PhysicalDomain=network_engine_domain  SubClassName=ps_input  LeftPortType=input  RightPortType=output  PseudoPeriodic=off  Frequencies=[]  NoiseDistribution=none  NoiseParameters=[]  Unit=W/(m^2*K)  AffineConversion=off  FilteringAndDerivatives=zero  SimscapeFilterOrder=1  InputFilterTimeConstant=1  UdotUserProvided=1
  Simulink-PS Converter2 : nesl_utility/Simulink-PS Converter  PhysicalDomain=network_engine_domain  SubClassName=ps_input  LeftPortType=input  RightPortType=output  PseudoPeriodic=off  Frequencies=[]  NoiseDistribution=none  NoiseParameters=[]  Unit=K  AffineConversion=on  FilteringAndDerivatives=zero  SimscapeFilterOrder=1  InputFilterTimeConstant=1  UdotUserProvided=1
  Thermal Reference : fl_lib/Thermal/Thermal Elements/Thermal Reference
  T : PMIOPort  Side=Right
  C : PMIOPort  Port=2  Side=Right
  HC : PMIOPort  Port=3  Side=Right
  wires:
  Saturation/1 -> Fcn/1
  Product1/1 -> C_air/1  "mdot_air"
  Constant4/1 -> Product/2
  Constant2/1 -> Product1/2
  Product/1 -> Product1/1
  C_air/1 -> Simulink-PS Converter/1
  Constant1/1 -> C_air/2
  T_air/1 -> Simulink-PS Converter2/1
  MinMax/1 -> Simulink-PS Converter1/1
  Constant5/1 -> MinMax/2
  Product2/1 -> MinMax/1
  Fcn/1 -> Product2/1
  Divide/1 -> Saturation/1
  Constant3/1 -> Product2/2
  Constant/1 -> Divide/2
  V_air/1 -> Divide/1, Product/1
  connections:
  Ideal Temperature Source/LConn1 -- T/RConn1
  Simulink-PS Converter2/RConn1 -- Ideal Temperature Source/RConn1
  Thermal Reference/LConn1 -- Ideal Temperature Source/RConn2
  Simulink-PS Converter1/RConn1 -- HC/RConn1
  C/RConn1 -- Simulink-PS Converter/RConn1
